simulink model "localmemory"  (R2017a)
settings: Solver=VariableStepAuto  StartTime=0.0  StopTime=10.0  RelTol=1e-3
settings Model: Creator=ptracton  LastModifiedBy=ptracton

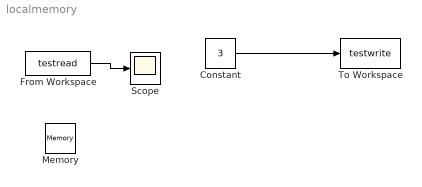
== system localmemory ==
  Constant : Constant  Value=3
  From Workspace : FromWorkspace  VariableName=testread  SampleTime=0
  Memory : Memory
  Scope : Scope
  To Workspace : ToWorkspace  VariableName=testwrite  SaveFormat=Timeseries  SampleTime=-1
  wires:
  Constant/1 -> To Workspace/1
  From Workspace/1 -> Scope/1
